simulink subsystem "Day2_Scenario_2_3"  (R2024a)
settings: Solver=VariableStepAuto  StartTime=0.0  StopTime=10.0  RelTol=1e-3
libraries: CarMaker4SL x6
settings Model: Creator=junhyung.cha  LastModifiedBy=User

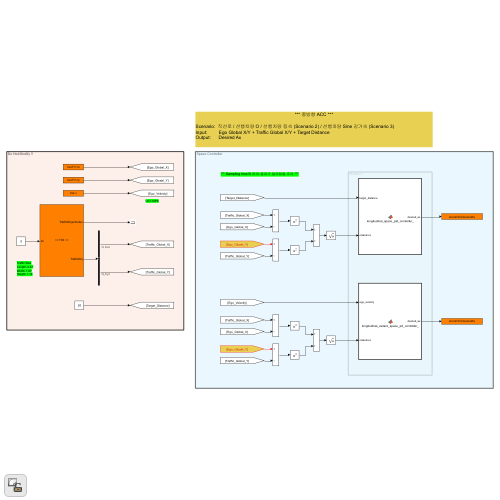
[thumbnail: Simulink's stored preview of the top-level diagram]
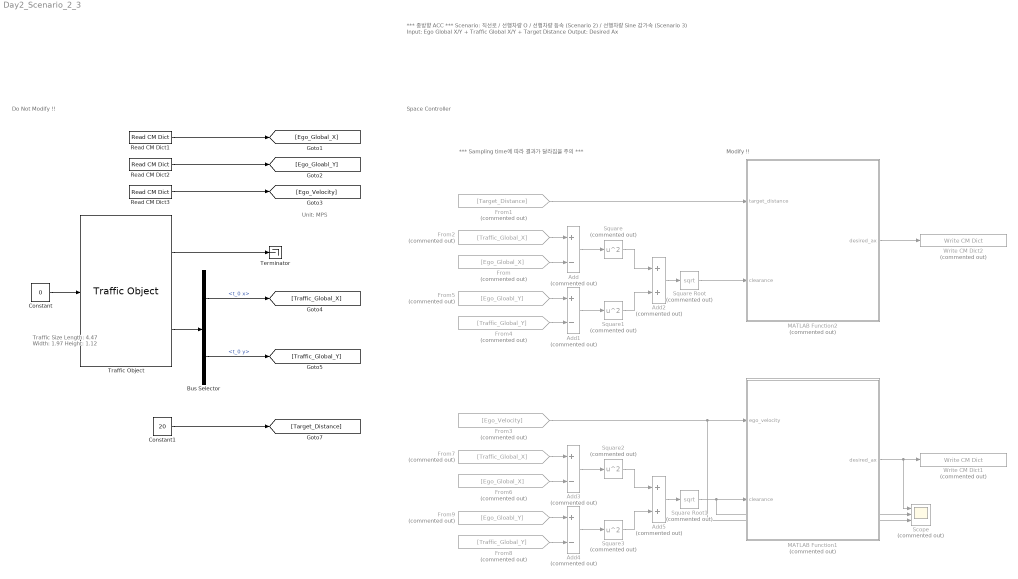
== system Day2_Scenario_2_3 ==
  note: *** Sampling time에 따라 결과가 달라짐을 주의 ***
  note: Space Controller
  note: Modify !!
  note: Do Not Modify !!
  note: Traffic Size
      | Length: 4.47
      | Width: 1.97
      | Height: 1.12
  note: *** 종방향 ACC ***
      |
      | Scenario: 직선로 / 선행차량 O / 선행차량 등속 (Scenario 2) / 선행차량 Sine 감가속 (Scenario 3)
      | Input: Ego Global X/Y + Traffic Global X/Y + Target Distance
      | Output: Desired Ax
  note: Unit: MPS
  Add{,1,3..4} (4 alike) : Sum  Commented=on  Inputs=+-
  Add2 : Sum  Commented=on
  Add5 : Sum  Commented=on
  Bus Selector : BusSelector  OutputSignals=t_0 x,t_0 y
  Constant : Constant  Value=0
  Constant1 : Constant  Value=20
  From : From  Commented=on  GotoTag=Ego_Global_X
  From1 : From  Commented=on  GotoTag=Target_Distance
  From2 : From  Commented=on  GotoTag=Traffic_Global_X
  From3 : From  Commented=on  GotoTag=Ego_Velocity
  From4 : From  Commented=on  GotoTag=Traffic_Global_Y
  From5 : From  Commented=on  GotoTag=Ego_Gloabl_Y
  From6 : From  Commented=on  GotoTag=Ego_Global_X
  From7 : From  Commented=on  GotoTag=Traffic_Global_X
  From8 : From  Commented=on  GotoTag=Traffic_Global_Y
  From9 : From  Commented=on  GotoTag=Ego_Gloabl_Y
  MATLAB Function1 : MATLAB Function  Commented=on  TreatAsAtomicUnit=on
  MATLAB Function2 : MATLAB Function  Commented=on  TreatAsAtomicUnit=on
  Read CM Dict1 : CarMaker4SL/Read CM Dict  xname=Car.Fr1.tx  xsync=off  xstime=Inherited
  Read CM Dict2 : CarMaker4SL/Read CM Dict  xname=Car.Fr1.ty  xsync=off  xstime=Inherited
  Read CM Dict3 : CarMaker4SL/Read CM Dict  xname=Car.v  xsync=off  xstime=Inherited
  Scope : Scope  Commented=on  NumInputPorts=3
  Square{,1..3} (4 alike) : Math  Commented=on  Operator=square
  Square Root : Sqrt  Commented=on
  Square Root1 : Sqrt  Commented=on
  Terminator : Terminator
  Traffic Object : CarMaker4SL/Traffic Object  xname=T00  ximode=Traffic Id  xstime=Inherited
      settings: SourceProductName=CarMaker4SL
  Write CM Dict1 : CarMaker4SL/Write CM Dict  Commented=on  xname=AccelCtrl.DesiredAx  xsync=off
  Write CM Dict2 : CarMaker4SL/Write CM Dict  Commented=on  xname=AccelCtrl.DesiredAx  xsync=off
  wires:
  Read CM Dict2/1 -> [Ego_Gloabl_Y]
  MATLAB Function2/1(desired_ax) -> Write CM Dict2/1
  Read CM Dict1/1 -> [Ego_Global_X]
  Constant/1 -> Traffic Object/1
  Traffic Object/2 -> Bus Selector/1
  Traffic Object/1 -> Terminator/1
  Bus Selector/1 -> [Traffic_Global_X]  "<t_0 x>"
  Bus Selector/2 -> [Traffic_Global_Y]  "<t_0 y>"
  Square Root/1 -> MATLAB Function2/2(clearance)
  Constant1/1 -> [Target_Distance]
  From/1 -> Add/2
  From2/1 -> Add/1
  From4/1 -> Add1/2
  From5/1 -> Add1/1
  Add1/1 -> Square1/1
  Add2/1 -> Square Root/1
  Square/1 -> Add2/1
  Square1/1 -> Add2/2
  From1/1 -> MATLAB Function2/1(target_distance)
  Add/1 -> Square/1
  Read CM Dict3/1 -> [Ego_Velocity]
  From3/1 -> MATLAB Function1/1(ego_velocity), Scope/3
  Add3/1 -> Square2/1
  Square3/1 -> Add5/2
  Square2/1 -> Add5/1
  Add5/1 -> Square Root1/1
  Add4/1 -> Square3/1
  From9/1 -> Add4/1
  From8/1 -> Add4/2
  From7/1 -> Add3/1
  From6/1 -> Add3/2
  Square Root1/1 -> MATLAB Function1/2(clearance), Scope/2
  MATLAB Function1/1(desired_ax) -> Write CM Dict1/1, Scope/1

== matlab function Day2_Scenario_2_3/MATLAB Function1 ==
  settings: updateMethod=DISCRETE  sampleTime=0.05
  data: ego_velocity input; desired_ax output; clearance input
function desired_ax = longitudinal_variant_space_pd_controller_(ego_velocity, clearance)
    % Controller parameters
    time_gap = 1.5;    % [s] desired time gap
    min_distance = 5;  % [m] minimum distance (stop case)

    Kp = 0.5;  % Proportional gain
    Kd = 0.3;  % Derivative gain

    % Compute dynamic target distance based on ego speed
    target_distance = max(time_gap * ego_velocity, min_distance);  % prevent zero target

    % Compute error
    error = clearance - target_distance;

    % Derivative term using persistent variable
    persistent prev_error;
    if isempty(prev_error)
        prev_error = error;
    end

    % Time step (assuming fixed)
    dt = 0.05;  % [s] 50 ms

    % Derivative of error
    derivative = (error - prev_error) / dt;

    % PD control output
    desired_ax = Kp * error + Kd * derivative;

    % Clamp acceleration (optional)
    desired_ax = max(min(desired_ax, 3.0), -5.0);  % [m/s^2]

    % Update previous error
    prev_error = error;
end

== matlab function Day2_Scenario_2_3/MATLAB Function2 ==
  settings: updateMethod=DISCRETE  sampleTime=0.05
  data: target_distance input; desired_ax output; clearance input
function desired_ax = longitudinal_space_pid_controller_(target_distance, clearance)
    %desired_ax = 0;
    % longitudinal_space_pid_controller_
%   Inputs:
%     target_distance - 목표 간격 [m]
%     clearance       - 현재 간격     [m]
%   Output:
%     desired_ax      - 명령 종방향 가속도 [m/s^2]

  %#codegen
  persistent Kp Ki Kd dt prev_error integral
  if isempty(Kp)
    % — 튜닝 파라미터 —
    Kp = 0.8;    % 비례 이득
    Ki = 0.001;    % 적분 이득
    Kd = 0.99;   % 미분 이득
    dt = 0.1;    % 제어 주기 [s]
    % — 초기화 —
    prev_error = target_distance - clearance;
    integral   = 0;
  end

  % 1) 오차 계산
  error = target_distance-clearance;
  % 2) 적분 업데이트
  integral = integral + error * dt;
  % 3) 미분 계산
  derivative = (error - prev_error) / dt;
  % 4) PID 법칙
  desired_ax = -(Kp * error + Ki * integral + Kd * derivative);
  % 5) 상태 저장
  prev_error = error;
end
